simulink model "successfulSaturation_decoderN4"  (R2016b)
settings: Solver=FixedStepDiscrete  StartTime=0.0  StopTime=10.0  RelTol=1e-3
settings Model: DataTypeOverride=Off  Creator=hasee  LastModifiedBy=hasee
settings DataIOCC: LimitDataPoints=on  SaveOutput=off  SaveTime=off
settings OptimizationCC: BlockReduction=off  ConditionallyExecuteInputs=off  DefaultParameterBehavior=Inlined  LifeSpan=inf
settings DebuggingCC: AlgebraicLoopMsg=error  SingleTaskRateTransMsg=error  AllowSymbolicDim=off  StrictBusMsg=ErrorOnBusTreatedAsVector  SFUnexpectedBacktrackingDiag=warning  SFNoUnconditionalDefaultTransitionDiag=warning  SFExecutionAtInitializationDiag=none
settings HardwareCC: ProdBitPerPointer=32  ProdBitPerSizeT=32  ProdBitPerPtrDiffT=32  ProdLargestAtomicFloat=None  ProdIntDivRoundTo=Undefined  ProdEndianess=Unspecified  ProdWordSize=32  ProdHWDeviceType=ASIC/FPGA->ASIC/FPGA  ProdEqTarget=off
settings GRTTargetCC: TargetLangStandard=C89/C90 (ANSI)  GeneratePreprocessorConditionals=Disable all
settings ConfigComp: CovScope=ReferencedModels  CovMetricSettings=dw  CovHtmlReporting=on  CovSaveCumulativeToWorkspaceVar=on  CovSaveSingleToWorkspaceVar=on  CovExternalEMLEnable=off  CovSFcnEnable=off

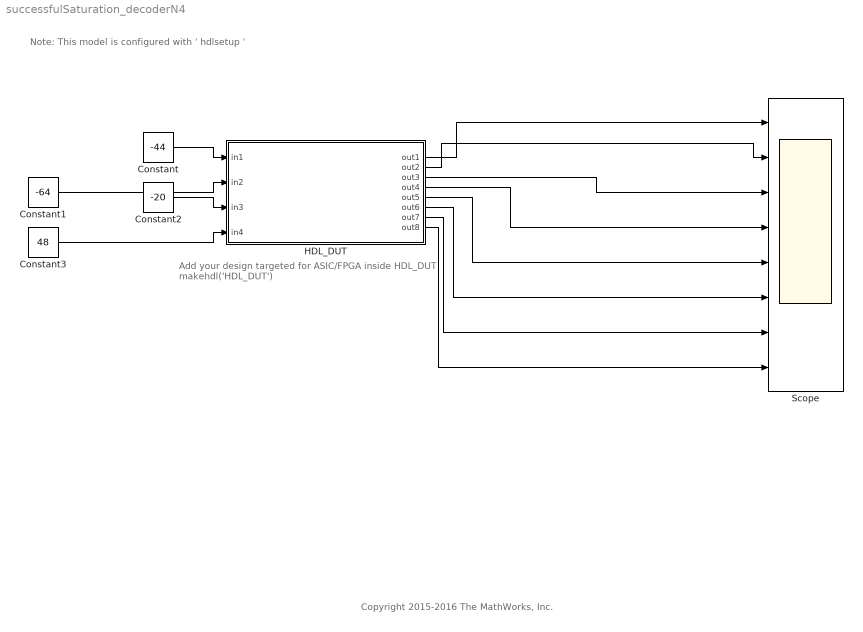
== system successfulSaturation_decoderN4 ==
  note: Note: This model is configured with ' hdlsetup '
  note: Add your design targeted for ASIC/FPGA inside HDL_DUT
      | makehdl('HDL_DUT')
  note: Copyright 2015-2016 The MathWorks, Inc.
  Constant : Constant  Value=-44  OutDataTypeStr=int8  SampleTime=-1
  Constant1 : Constant  Value=-64  OutDataTypeStr=int8  SampleTime=-1
  Constant2 : Constant  Value=-20  OutDataTypeStr=int8  SampleTime=-1
  Constant3 : Constant  Value=48  OutDataTypeStr=int8  SampleTime=-1
  HDL_DUT : Subsystem
  Scope : Scope  NumInputPorts=8
  wires:
  Constant/1 -> HDL_DUT/1(in1)
  Constant1/1 -> HDL_DUT/2(in2)
  HDL_DUT/1(out1) -> Scope/1
  HDL_DUT/2(out2) -> Scope/2
  HDL_DUT/3(out3) -> Scope/3
  Constant2/1 -> HDL_DUT/3(in3)
  Constant3/1 -> HDL_DUT/4(in4)
  HDL_DUT/4(out4) -> Scope/4
  HDL_DUT/5(out5) -> Scope/5
  HDL_DUT/6(out6) -> Scope/6
  HDL_DUT/7(out7) -> Scope/7
  HDL_DUT/8(out8) -> Scope/8

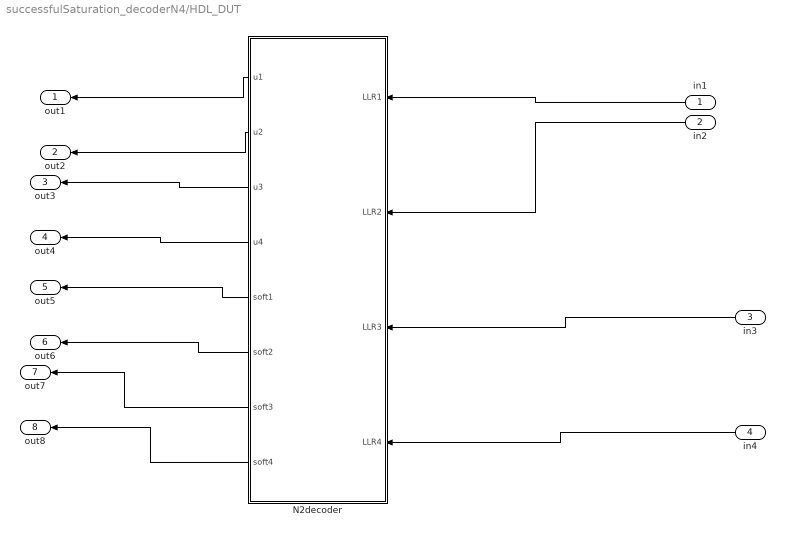
== system successfulSaturation_decoderN4/HDL_DUT ==
  in1 : Inport
  in2 : Inport  Port=2
  in3 : Inport  Port=3
  in4 : Inport  Port=4
  N2decoder : MATLAB Function  TreatAsAtomicUnit=on
  out1 : Outport
  out2 : Outport  Port=2
  out3 : Outport  Port=3
  out4 : Outport  Port=4
  out5 : Outport  Port=5
  out6 : Outport  Port=6
  out7 : Outport  Port=7
  out8 : Outport  Port=8
  wires:
  N2decoder/1(u1) -> out1/1
  N2decoder/2(u2) -> out2/1
  in4/1 -> N2decoder/4(LLR4)
  N2decoder/4(u4) -> out4/1
  N2decoder/5(soft1) -> out5/1
  N2decoder/6(soft2) -> out6/1
  N2decoder/3(u3) -> out3/1
  N2decoder/7(soft3) -> out7/1
  N2decoder/8(soft4) -> out8/1
  in1/1 -> N2decoder/1(LLR1)
  in2/1 -> N2decoder/2(LLR2)
  in3/1 -> N2decoder/3(LLR3)

== matlab function successfulSaturation_decoderN4/HDL_DUT/N2decoder ==
  data: LLR1 input; u1 output; u2 output; u3 output; u4 output; soft1 output; LLR2 input; LLR3 input; LLR4 input; soft2 output; soft3 output; soft4 output
function [u1,u2,u3,u4,soft1,soft2,soft3,soft4] = fcn(LLR1,LLR2,LLR3,LLR4)
%状态机默认状态是S1（为0）
%每个输出都需要在每一个case里面定义值，或者一开始就定义初值。
%思路：全部状态机操作的都是reg，到最后一个状态的时候统一把所有output都输出reg里面的值，在此之前output可以都为0；
persistent state_reg;
persistent LLR1_reg;
persistent LLR2_reg;
persistent LLR3_reg;
persistent LLR4_reg;
persistent L21y12_reg;
persistent L21y34_reg;
persistent L41y14_reg;
persistent L42y14u11_reg;
persistent L22y12u12_reg;
persistent L22y34u2_reg;
persistent L43y14u12_reg;
persistent L44y14u13_reg;

persistent u1_reg;
persistent soft1_reg;
persistent u2_reg;
persistent soft2_reg;
persistent u3_reg;
persistent soft3_reg;
persistent u4_reg;
persistent soft4_reg;


if isempty(state_reg)
    state_reg = fi(0, 0, 3, 0, hdlfimath);
    LLR1_reg=  LLR1;
    LLR2_reg=  LLR2;
    LLR3_reg=  LLR3;
    LLR4_reg=  LLR4;
    %初始化计算u1需要的LLR
    L21y12_reg=int8(0);
    L21y34_reg=int8(0);
    L41y14_reg=int8(0);
    %初始化计算u2需要的LLR
    L42y14u11_reg=int8(0);
    %初始化计算u3需要的LLR
    L22y12u12_reg=int8(0);
    L22y34u2_reg = int8(0);
    L43y14u12_reg = int8(0);
    L44y14u13_reg = int8(0);

    %初始化计算u4需要的LLR
    %u4所需要的前面都已经计算好了
    
    
    %初始化output的寄存器
    u1_reg=false;
    soft1_reg=int8(0);
    u2_reg=false;
    soft2_reg=int8(0);
    u3_reg=false;
    soft3_reg=int8(0);
    u4_reg=false;
    soft4_reg=int8(0);
end

S1 = 0;
S2 = 1;
S3 = 2;
S4 = 3;
S5 = 4;

soft1=soft1_reg;
u1=u1_reg;
soft2=soft2_reg;
u2=u2_reg;
soft3=soft3_reg;
u3=u3_reg;
soft4=soft4_reg;
u4=u4_reg;

%有限状态机
switch (state_reg)
    case S1
        L21y12_reg=f(LLR1_reg,LLR2_reg);
        L21y34_reg=f(LLR3_reg,LLR4_reg);
        state_reg(1) = S2;
    case S2
        L41y14_reg=f(L21y12_reg,L21y34_reg);
        soft1_reg=L41y14_reg;
        u1_reg=decide(soft1,1);
        state_reg(1) = S3;
    case S3
        L42y14u11_reg=g(L21y12_reg,L21y34_reg,u1_reg);
        soft2_reg=L42y14u11_reg;
        u2_reg=decide(soft2_reg,2);
        state_reg(1) = S4;
    case S4
        L22y12u12_reg=g(LLR1_reg,LLR2_reg,xor(u1_reg,u2_reg));
        L22y34u2_reg = g(LLR3_reg,LLR4_reg,u2_reg);
        L43y14u12_reg=f(L22y12u12_reg,L22y34u2_reg);
        soft3_reg=L43y14u12_reg;
        u3_reg=decide(soft3_reg,3);
        state_reg(1) = S5;
    case S5
        L44y14u13_reg = g(L22y12u12_reg,L22y34u2_reg,u3_reg);
        soft4_reg=L44y14u13_reg;
        u4_reg=decide(soft4_reg,4);
end



%判定输出u函数开始；根据软信息和冻结比特位信息；FZlookup是冻结比特位置信息，false代表这一位是冻结比特
function out = decide(soft,position)
persistent FZlookup;
if isempty(FZlookup)
    FZlookup = [false;false;true;true];
end
if FZlookup(position) == true
    if soft > 0  %PCparams.LLR(1) 就是根据最左边的LLR硬裁决
        out = false;
    else
        out = true;
    end
else
    out =FZlookup(position);
end%判定输出u函数结束


function out = f(in1,in2)
%f函数开始
if (in1>0 && in2>0) ||(in1<0 && in2<0)
    out=min(abs(in1),abs(in2));
    %f函数当符号为正时结束
else
    out=-min(abs(in1),abs(in2));
    %f函数当符号为负时结束
end


function out = g(in1,in2,b)
%g函数开始
 if (b == 0)
     out=in1 + in2;
     %g函数当b==0时结束
 else
     out=-in1 + in2;
     %g函数当b==1时结束
end
